simulink model "maglev_preliminary"  (R2024a)
settings: Solver=VariableStepAuto  StartTime=0.0  StopTime=10.0  RelTol=1e-3
values from neighbouring files (symbols this model uses):
  m = 0.06157    [init.m]
undefined symbols (not defined in the file or in its folder): kv, L, R
settings Model: Creator=User  LastModifiedBy=Bocchio
settings DebuggingCC: UnconnectedInputMsg=warning  UnconnectedOutputMsg=warning  UnconnectedLineMsg=warning
settings ModelReferenceCC: EnableRefExpFcnMdlSchedulingChecks=on
settings RTWCC: GPUComputeCapability=3.5  DLArmComputeVersion=19.05

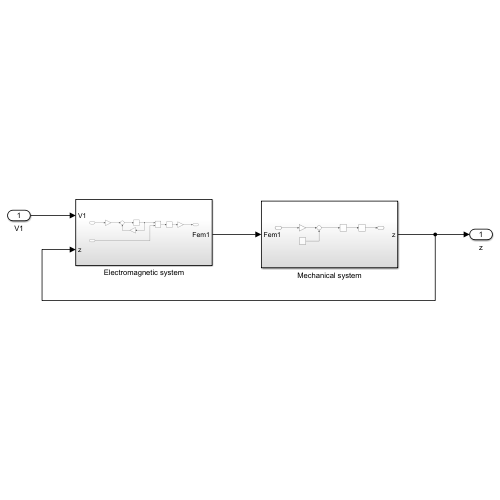
[thumbnail: Simulink's stored preview of the top-level diagram]
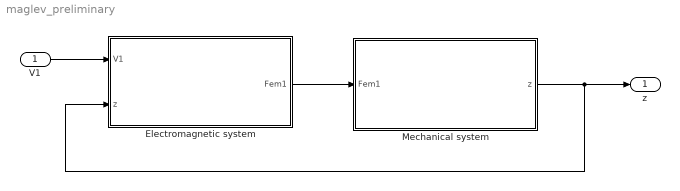
== system maglev_preliminary ==
  V1 : Inport
  Electromagnetic system : Subsystem
  Mechanical system : Subsystem
  z : Outport
  wires:
  V1/1 -> Electromagnetic system/1(V1)
  Mechanical system/1(z) -> z/1, Electromagnetic system/2(z)
  Electromagnetic system/1(Fem1) -> Mechanical system/1(Fem1)

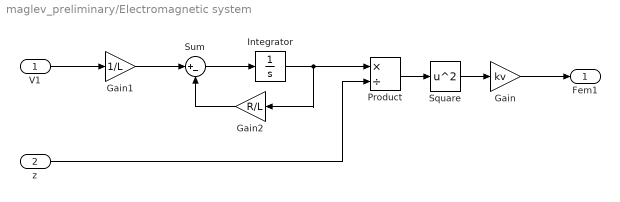
== system maglev_preliminary/Electromagnetic system ==
  V1 : Inport
  z : Inport  Port=2
  Gain : Gain  Gain=kv
  Gain1 : Gain  Gain=1/L
  Gain2 : Gain  Gain=R/L
  Integrator : Integrator
  Product : Product  Inputs=*/
  Square : Math  Operator=square
  Sum : Sum  Inputs=|+-
  Fem1 : Outport
  wires:
  Gain/1 -> Fem1/1
  z/1 -> Product/2
  Square/1 -> Gain/1
  Product/1 -> Square/1
  Integrator/1 -> Product/1, Gain2/1
  V1/1 -> Gain1/1
  Gain1/1 -> Sum/1
  Gain2/1 -> Sum/2
  Sum/1 -> Integrator/1

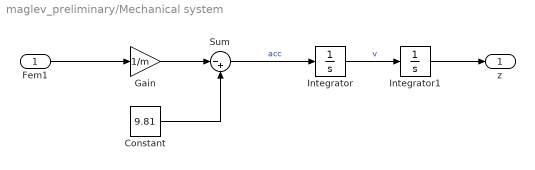
== system maglev_preliminary/Mechanical system ==
  Fem1 : Inport
  Constant : Constant  Value=9.81
  Gain : Gain  Gain=1/m
  Integrator : Integrator
  Integrator1 : Integrator  InitialCondition=0.02
  Sum : Sum  Inputs=|-+
  z : Outport
  wires:
  Fem1/1 -> Gain/1
  Gain/1 -> Sum/1
  Constant/1 -> Sum/2
  Sum/1 -> Integrator/1  "acc"
  Integrator/1 -> Integrator1/1  "v"
  Integrator1/1 -> z/1
